simulink model "REALTIME_PART1_feedforward"  (R2020b)
settings: Solver=ode3  StartTime=0.0  StopTime=9  FixedStep=0.001  RelTol=1e-3
undefined symbols (not defined in the file): BEMF_comp, Beq_hat, ctrl, degs2rpm, denHwa, denHws, friction_comp, gbox, inertia_comp, National_Instruments, numHwa, numHws, PCI, rpm2rads, sens, tau_hat
libraries: sldrtlib x2, simulink x1
settings Model: ExtModeTrigDuration=10000  Creator=gioel  LastModifiedBy=ambrosingi
settings DataIOCC: ReturnWorkspaceOutputs=off
settings RTWCC: Description=Simulink Desktop Real-Time  SystemTargetFile=sldrt.tlc  TemplateMakefile=sldrt.tmf  RTWCompilerOptimization=on
settings CodeAppCC: MaxIdLength=95
settings SimulinkDesktopRealTimeCC: TargetPreCompLibLocation=C:\Program Files\MATLAB\R2020b\toolbox\sldrt\lib\win64

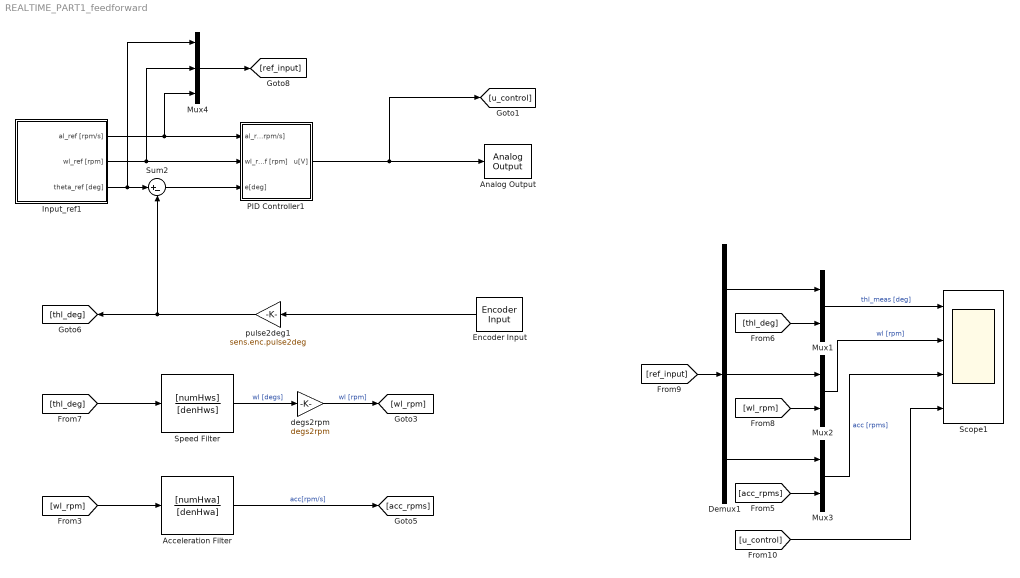
== system REALTIME_PART1_feedforward ==
  Acceleration Filter : TransferFcn  Numerator=[numHwa]  Denominator=[denHwa]
  Analog Output : sldrtlib/Analog Output  SampleTime=0.001  MaxMissedTicks=10  ShowMissedTicks=off  YieldWhenWaiting=off  DrvName=National_Instruments/PCI-6221  DrvAddress=4294967295  DrvOptions=[0 0 0 2 0]  Channels=1  RangeMode=1  VoltRange=1  InitialValue=0  FinalValue=0
      settings: AttributesFormatString=National Instruments\nPCI-6221 [auto]
  Demux1 : Demux  Outputs=3
  Encoder Input : sldrtlib/Encoder Input  SampleTime=0.001  MaxMissedTicks=10  ShowMissedTicks=off  YieldWhenWaiting=off  DrvName=National_Instruments/PCI-6221  DrvAddress=4294967295  DrvOptions=[0 0 0 2 0]  Channels=1  QuadMode=3  IndexPulse=1  InputFilter=Inf  DataType=1
      settings: AttributesFormatString=National Instruments\nPCI-6221 [auto]
  Input_ref1 : Subsystem
  Mux1 : Mux  Inputs=2
  Mux2 : Mux  Inputs=2
  Mux3 : Mux  Inputs=2
  Mux4 : Mux  Inputs=3
  PID Controller1 : Subsystem
  Scope1 : Scope  NumInputPorts=4
  Speed Filter : TransferFcn  Numerator=[numHws]  Denominator=[denHws]
  Sum2 : Sum  Inputs=|+-
  degs2rpm : Gain  Gain=degs2rpm
  pulse2deg1 : Gain  Gain=sens.enc.pulse2deg
  wires:
  pulse2deg1/1 -> [thl_deg], Sum2/2
  Encoder Input/1 -> pulse2deg1/1
  degs2rpm/1 -> [wl_rpm]  "wl [rpm]"
  PID Controller1/1(u[V]) -> Analog Output/1, [u_control]
  Input_ref1/3(theta_ref [deg]) -> Mux4/1, Sum2/1
  Speed Filter/1 -> degs2rpm/1  "wl [degs]"
  Acceleration Filter/1 -> [acc_rpms]  "acc[rpm/s]"
  [wl_rpm] -> Acceleration Filter/1
  [u_control] -> Scope1/4
  Mux3/1 -> Scope1/3  "acc [rpms]"
  [thl_deg] -> Mux1/2
  [thl_deg] -> Speed Filter/1
  Mux1/1 -> Scope1/1  "thl_meas [deg]"
  Input_ref1/1(al_ref [rpm/s]) -> PID Controller1/1("al_ref [rpm/s]  "), Mux4/3
  Input_ref1/2(wl_ref [rpm]) -> PID Controller1/2("wl_ref [rpm] "), Mux4/2
  [wl_rpm] -> Mux2/2
  [acc_rpms] -> Mux3/2
  Mux4/1 -> [ref_input]
  [ref_input] -> Demux1/1
  Sum2/1 -> PID Controller1/3(e[deg])
  Mux2/1 -> Scope1/2  "wl [rpm]"
  Demux1/1 -> Mux1/1
  Demux1/2 -> Mux2/1
  Demux1/3 -> Mux3/1

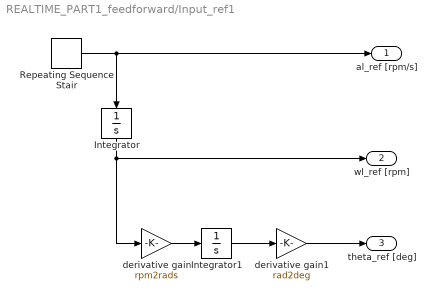
== system REALTIME_PART1_feedforward/Input_ref1 ==
  Integrator : Integrator
  Integrator1 : Integrator
  Repeating Sequence Stair : simulink/Sources/Repeating Sequence Stair  OutValues=[900 0 -900 -900 0 900].'  tsamp=0.5  OutMin=[]  OutMax=[]  OutDataTypeStr=double  OutputDataTypeScalingMode=double  OutDataType=fixdt(0,8)  ConRadixGroup=Best Precision: Vector-wise  OutScaling=2^-12
  derivative gain : Gain  Gain=rpm2rads
  derivative gain1 : Gain  Gain=rad2deg
  al_ref [rpm/s] : Outport  VectorParamsAs1DForOutWhenUnconnected=off
  wl_ref [rpm] : Outport  Port=2  VectorParamsAs1DForOutWhenUnconnected=off
  theta_ref [deg] : Outport  Port=3  VectorParamsAs1DForOutWhenUnconnected=off
  wires:
  Integrator/1 -> derivative gain/1, wl_ref [rpm]/1
  derivative gain/1 -> Integrator1/1
  derivative gain1/1 -> theta_ref [deg]/1
  Integrator1/1 -> derivative gain1/1
  Repeating Sequence Stair/1 -> Integrator/1, al_ref [rpm/s]/1

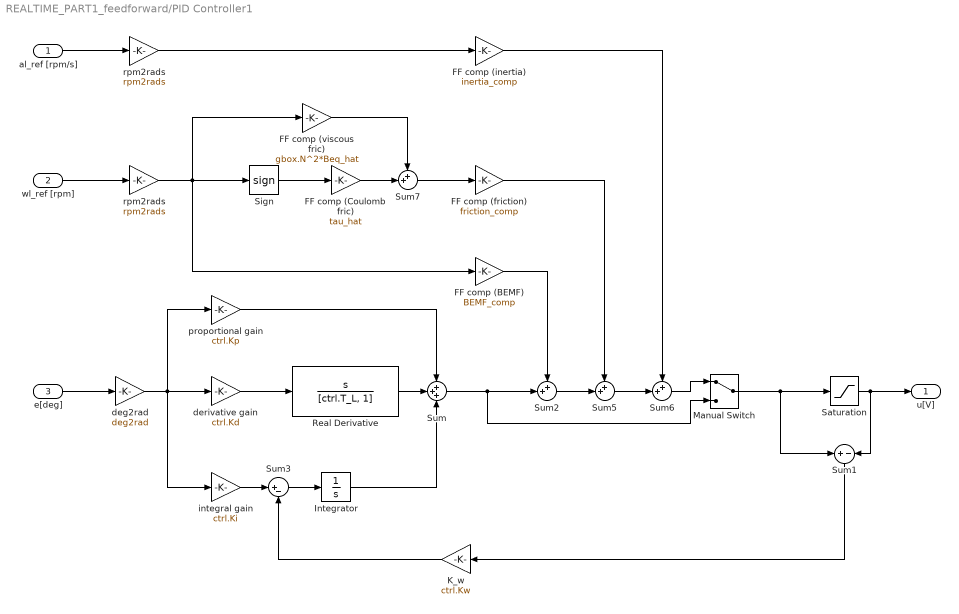
== system REALTIME_PART1_feedforward/PID Controller1 ==
  "al_ref [rpm/s]  " : Inport
  "wl_ref [rpm] " : Inport  Port=2
  e[deg] : Inport  Port=3
  FF comp (Coulomb fric) : Gain  Gain=tau_hat
  FF comp (viscous fric) : Gain  Gain=gbox.N^2*Beq_hat
  FF comp (BEMF) : Gain  Gain=BEMF_comp
  FF comp (friction) : Gain  Gain=friction_comp
  FF comp (inertia) : Gain  Gain=inertia_comp
  Integrator : Integrator
  K_w : Gain  Gain=ctrl.Kw
  Manual Switch : ManualSwitch
  Real Derivative : TransferFcn  Numerator=[1 0]  Denominator=[ctrl.T_L, 1]
  Saturation : Saturate  UpperLimit=10  LowerLimit=-10
  "Sign " : Signum  ZeroCross=off
  Sum : Sum  Inputs=+++
  Sum1 : Sum  Inputs=+|-
  Sum{2,5..7} (4 alike) : Sum  Inputs=++|
  Sum3 : Sum  Inputs=|+-
  deg2rad : Gain  Gain=deg2rad
  derivative gain : Gain  Gain=ctrl.Kd
  integral gain : Gain  Gain=ctrl.Ki
  proportional gain : Gain  Gain=ctrl.Kp
  rpm2rads : Gain  Gain=rpm2rads
  "rpm2rads " : Gain  Gain=rpm2rads
  u[V] : Outport
  wires:
  Manual Switch/1 -> Saturation/1, Sum1/1
  Sum6/1 -> Manual Switch/1
  FF comp (inertia)/1 -> Sum6/1
  FF comp (friction)/1 -> Sum5/1
  FF comp (BEMF)/1 -> Sum2/1
  "wl_ref [rpm] "/1 -> "rpm2rads "/1
  e[deg]/1 -> deg2rad/1
  "al_ref [rpm/s]  "/1 -> rpm2rads/1
  Sum/1 -> Sum2/2, Manual Switch/2
  "rpm2rads "/1 -> "Sign "/1, FF comp (viscous fric)/1, FF comp (BEMF)/1
  "Sign "/1 -> FF comp (Coulomb fric)/1
  rpm2rads/1 -> FF comp (inertia)/1
  FF comp (viscous fric)/1 -> Sum7/1
  FF comp (Coulomb fric)/1 -> Sum7/2
  Sum2/1 -> Sum5/2
  Sum7/1 -> FF comp (friction)/1
  Sum5/1 -> Sum6/2
  K_w/1 -> Sum3/2
  Sum3/1 -> Integrator/1
  integral gain/1 -> Sum3/1
  Integrator/1 -> Sum/3
  deg2rad/1 -> proportional gain/1, derivative gain/1, integral gain/1
  derivative gain/1 -> Real Derivative/1
  Sum1/1 -> K_w/1
  proportional gain/1 -> Sum/1
  Real Derivative/1 -> Sum/2
  Saturation/1 -> u[V]/1, Sum1/2
